simulink model "RightTrajectoryAgent"  (Simulink 6.5)
settings: Solver=ode45  SolverMode=SingleTasking  StartTime=0.0  StopTime=10.0  RelTol=1e-3  AbsTol=1e-6
settings Model: Creator=The MathWorks Inc.  LastModifiedBy=suarezjl  ExtModeTrigMode=oneshot  ExtModeArmWhenConnect=off  ExtModeAutoUpdateStatusClock=off
settings DataIOCC: LimitDataPoints=off  SignalLoggingName=logsOut
settings OptimizationCC: BooleanDataType=off  InlineInvariantSignals=on
settings DebuggingCC: CheckExecutionContextPreStartOutputMsg=on  CheckExecutionContextRuntimeOutputMsg=on  SolverPrmCheckMsg=none  MultiTaskDSMMsg=warning  MultiTaskCondExecSysMsg=none  IntegerOverflowMsg=none  StrictBusMsg=None
settings HardwareCC: TargetUnknown=on
settings ModelReferenceCC: UpdateModelReferenceTargets=IfOutOfDate
settings RTWCC: IncludeERTFirstTime=on

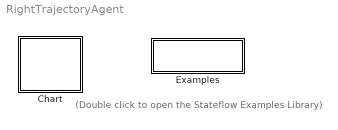
== system RightTrajectoryAgent ==
  note: (Double click to open the
      | Stateflow Examples Library)
  Chart : Stateflow chart
  Examples : Subsystem
      settings: OpenFcn=sf('Private','sf_examples')
      mask Display: disp('Examples')

== system RightTrajectoryAgent/Examples ==

== stateflow chart Chart ==
  state InitializeFunctions
    Hungerforce\CogDemo\RightTrajectoryAgent\LoadHomePosition.Initialize()
    Hungerforce\CogDemo\RightTrajectoryAgent\PlayCurrentTraj.Initialize()
    Hungerforce\CogDemo\RightTrajectoryAgent\LoadHomePosition.Write2VS()
  state CopyCurrentLocation
    Hungerforce\CogDemo\RightTrajectoryAgent\CopyGoalPosition.CopyRowVector()
    Hungerforce\CogDemo\RightTrajectoryAgent\CopyCurrentPosition.CopyCurrentVector()
  state GenerateCurrentTrajectory
    Hungerforce\CogDemo\RightTrajectoryAgent\GenerateCurrentTraj.GenerateTrajectory()
  state PlayCurrentTrajectory
    Hungerforce\CogDemo\RightTrajectoryAgent\PlayCurrentTraj.OutputTrajectory()
    Hungerforce\CogDemo\RightTrajectoryAgent\StateMachine.Wait(1000)
  state CopyHomeLocation
    Hungerforce\CogDemo\RightTrajectoryAgent\CopyHomePosition.CopyRowVector()
    Hungerforce\CogDemo\RightTrajectoryAgent\CopyCurrentPosition.CopyCurrentVector()
  state PlayHomeTrajectory
    Hungerforce\CogDemo\RightTrajectoryAgent\PlayCurrentTraj.OutputTrajectory()
  state GenerateHomeTrajectory
    Hungerforce\CogDemo\RightTrajectoryAgent\GenerateCurrentTraj.GenerateTrajectory()
  state Check that object is seen
    Hungerforce\CogDemo\RightTrajectoryAgent\GenerateCurrentTraj.CheckForObject()
  (default) -> InitializeFunctions : Start
  InitializeFunctions -> Check that object is seen : Always
  CopyCurrentLocation -> GenerateCurrentTrajectory : Always
  GenerateCurrentTrajectory -> PlayCurrentTrajectory : Always
  PlayHomeTrajectory -> CopyCurrentLocation : Signal="Next"
  PlayCurrentTrajectory -> CopyHomeLocation : Always
  GenerateHomeTrajectory -> PlayHomeTrajectory : Always
  CopyHomeLocation -> GenerateHomeTrajectory : Always
  Check that object is seen -> CopyCurrentLocation : Signal ="Next"
